simulink model "OQPSK"  (R2024a)
settings: Solver=ode45  StartTime=0.0  StopTime=100  RelTol=1e-3  EnableMultiTasking=on
undefined symbols (not defined in the file): get
libraries: simulink x2, commdigbbndpm3 x2, commchan3 x1, commsink2 x1, commrandsrc3 x1
settings Model: Creator=Ammar  LastModifiedBy=Hoàng IRyS
settings SolverCC: AlgebraicLoopSolver=TrustRegion
settings DataIOCC: LimitDataPoints=on  SaveFormat=Array  SignalLoggingSaveFormat=ModelDataLogs  ReturnWorkspaceOutputs=off
settings OptimizationCC: ExpressionDepthLimit=2147483647  LifeSpan=inf
settings DebuggingCC: UnderspecifiedInitializationDetection=Classic  MergeDetectMultiDrivingBlocksExec=none  SolverPrmCheckMsg=warning  FcnCallInpInsideContextMsg=warning  UnconnectedInputMsg=warning  UnconnectedOutputMsg=warning  UnconnectedLineMsg=warning  StateNameClashWarn=warning  SFUnexpectedBacktrackingDiag=warning  SFNoUnconditionalDefaultTransitionDiag=warning  SFExecutionAtInitializationDiag=none  ArithmeticOperatorsInVariantConditions=warning
settings HardwareCC: ProdBitPerPointer=32  ProdBitPerSizeT=32  ProdBitPerPtrDiffT=32  ProdLargestAtomicFloat=None  ProdIntDivRoundTo=Undefined  ProdEndianess=Unspecified  ProdWordSize=32  ProdHWDeviceType=32-bit Generic
settings ModelReferenceCC: PropagateSignalLabelsOutOfModel=off
settings SFSimCC: SimUseLocalCustomCode=off  CustomCodeUndefinedFunction=UseInterfaceOnly
settings RTWCC: RTWUseLocalCustomCode=off  GPUComputeCapability=3.5
settings CodeAppCC: StateflowObjectComments=on
settings GRTTargetCC: TargetLangStandard=C89/C90 (ANSI)  CombineOutputUpdateFcns=off  GRTInterface=on
settings ConfigComp: CovMetricSettings=dw  CovSaveCumulativeToWorkspaceVar=on  CovSaveSingleToWorkspaceVar=on  CovExternalEMLEnable=off

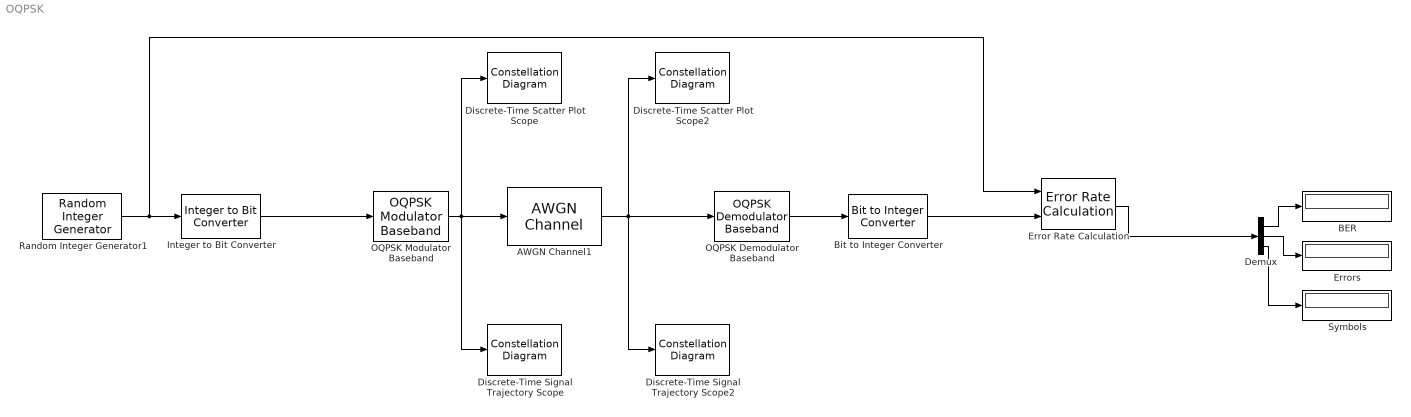
== system OQPSK ==
  AWGN Channel1 : commchan3/AWGN Channel  LegacyMode=on  NoiseMethod="Signal to noise ratio  (SNR)"  noiseMode="Signal to noise ratio  (Eb/No)"  EbNo=-10  EsNo=6  SNR=20  BitsPerSymbol=2  SignalPower=1  SamplesPerSymbol=1  SymbolPeriod=1/1000  VarianceSource=Parameter  Variance=1  RandomStream=Global stream  Seed=67  SimulateUsing=Code generation
  BER : Display
  Bit to Integer Converter : simulink/Logic and Bit Operations/Bit to Integer Converter  nbits=2  bitOrder=MSB first  signedOutputValues=Unsigned  outDtype=Inherit via internal rule  outDtypeSigned=Inherit via internal rule
      settings: LibrarySourceBlock=|
      | commutil2/Bit to Integer
      | Converter
  Demux : Demux  Outputs=3
  Discrete-Time Scatter Plot Scope : ConstellationDiagram  Tag=ScatterPlot  WindowPosition=[382.000000,84.000000,600.000000,600.000000,]  ScopeFrameLocation=window  FigPos=get(0,'defaultfigureposition');
  Discrete-Time Scatter Plot Scope2 : ConstellationDiagram  Tag=ScatterPlot  WindowPosition=[382.000000,84.000000,600.000000,600.000000,]  ScopeFrameLocation=window  FigPos=get(0,'defaultfigureposition');
  Discrete-Time Signal Trajectory Scope : ConstellationDiagram  Tag=SignalTrajectory  WindowPosition=[488.000000,242.000000,560.000000,420.000000,]  ScopeFrameLocation=window  SamplesPerSymbol=8  SymbolsToDisplaySource=on  SymbolsToDisplay=40  Title=Signal Trajectory  XLimits=1.5  YLimits=1.5  ShowTrajectory=on  ColorFading=on  FigPos=get(0,'defaultfigureposition');
  Discrete-Time Signal Trajectory Scope2 : ConstellationDiagram  Tag=SignalTrajectory  WindowPosition=[488.000000,242.000000,560.000000,420.000000,]  ScopeFrameLocation=window  SamplesPerSymbol=8  SymbolsToDisplaySource=on  SymbolsToDisplay=40  Title=Signal Trajectory  XLimits=1.5  YLimits=1.5  ShowTrajectory=on  ColorFading=on  FigPos=get(0,'defaultfigureposition');
  Error Rate Calculation : commsink2/Error Rate Calculation  N=1  st_delay=0  cp_mode=Entire frame  subframe=[]  PMode=Port  WsName=ErrorVec  RsMode2=off  stop=off  numErr=100  maxBits=1e6
  Errors : Display
  Integer to Bit Converter : simulink/Logic and Bit Operations/Integer to Bit Converter  nbits=2  signedInputValues=Unsigned  bitOrder=MSB first  outDtype=Inherit via internal rule
      settings: LibrarySourceBlock=|
      | commutil2/Integer to Bit
      | Converter
  OQPSK Demodulator Baseband : commdigbbndpm3/OQPSK Demodulator Baseband  OutType=Bit  Ph=0  Mapping=Gray  pulseShape=Custom  num=[0.7071 0.7071]  rolloff=0.2  filterSpan=10  sps=2  RateOptions=Enforce single-rate processing  outDtype2=double
  OQPSK Modulator Baseband : commdigbbndpm3/OQPSK Modulator Baseband  VariantControl=strcmp(pulseShape, 'Custom') && isequal(denom, 1)  InType=Bit  Mapping=Gray  Ph=0  pulseShape=Custom  num=[0.7071 0.7071]  denom=[1]  rolloff=0.2  filterSpan=10  sps=2  RateOptions=Enforce single-rate processing  outDtype=double  isIIR=off
  Random Integer Generator1 : commrandsrc3/Random Integer Generator  SetSize=2  SeedSource=Auto  Seed=0  SampleTime=1/1000  SamplesPerFrame=1  OutputDataType=double  SimulateUsing=Interpreted execution
  Symbols : Display
  wires:
  Demux/1 -> BER/1
  Demux/2 -> Errors/1
  Demux/3 -> Symbols/1
  Error Rate Calculation/1 -> Demux/1
  OQPSK Modulator Baseband/1 -> Discrete-Time Signal Trajectory Scope/1, Discrete-Time Scatter Plot Scope/1, AWGN Channel1/1
  AWGN Channel1/1 -> OQPSK Demodulator Baseband/1, Discrete-Time Signal Trajectory Scope2/1, Discrete-Time Scatter Plot Scope2/1
  Random Integer Generator1/1 -> Error Rate Calculation/1, Integer to Bit Converter/1
  Integer to Bit Converter/1 -> OQPSK Modulator Baseband/1
  Bit to Integer Converter/1 -> Error Rate Calculation/2
  OQPSK Demodulator Baseband/1 -> Bit to Integer Converter/1
